simulink model "mol2_5saturation"  (R2024b)
settings: Solver=VariableStepAuto  StartTime=0.0  StopTime=10.0  RelTol=1e-3
settings Model: Creator=24839  LastModifiedBy=24839

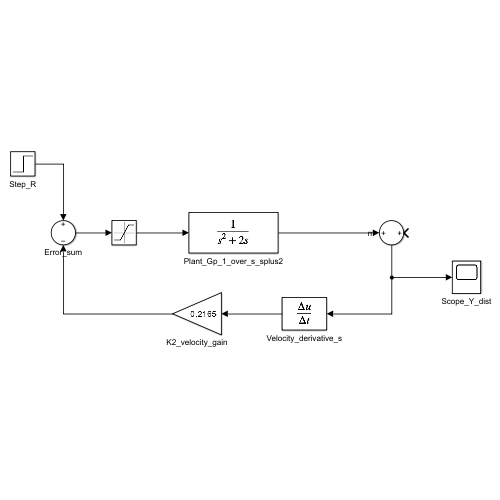
[thumbnail: Simulink's stored preview of the top-level diagram]
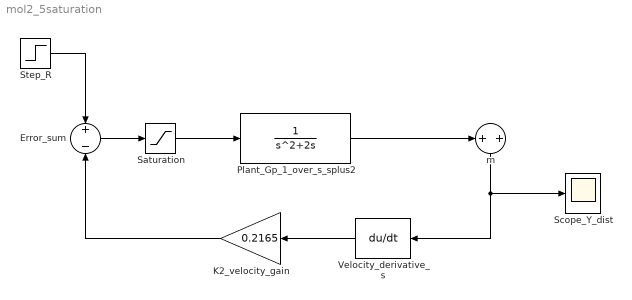
== system mol2_5saturation ==
  Error_sum : Sum  Inputs=+-
  K2_velocity_gain : Gain  Gain=0.2165
  Plant_Gp_1_over_s_splus2 : TransferFcn  Denominator=[1 2 0]
  Saturation : Saturate
  Scope_Y_dist : Scope
  Step_R : Step  Time=0  SampleTime=0
  Velocity_derivative_s : Derivative
  m : Sum
  wires:
  K2_velocity_gain/1 -> Error_sum/2
  Velocity_derivative_s/1 -> K2_velocity_gain/1
  m/1 -> Scope_Y_dist/1, Velocity_derivative_s/1
  Step_R/1 -> Error_sum/1
  Plant_Gp_1_over_s_splus2/1 -> m/1
  Error_sum/1 -> Saturation/1
  Saturation/1 -> Plant_Gp_1_over_s_splus2/1
